simulink model "Adddata_Model"  (R2023a)
settings: Solver=VariableStepAuto  StartTime=0.0  StopTime=10.0  RelTol=1e-3
libraries: NSA_DEVS_SINKS_ATOMIC x6, TimeSharedLib x3, NSA_DEVS_LOGISTICS_ATOMIC x2, NSA_DEVS_SOURCES_ATOMIC x1
settings Model: Creator=david  LastModifiedBy=peter

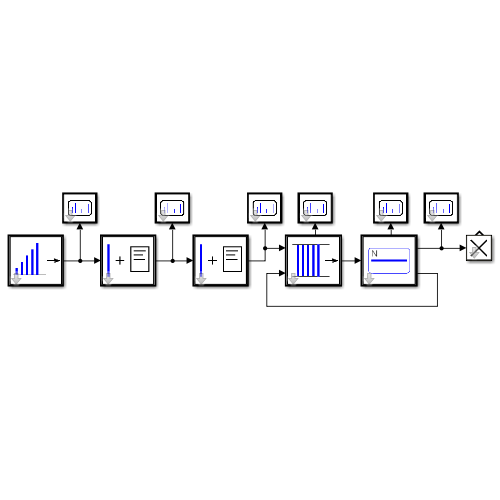
[thumbnail: Simulink's stored preview of the top-level diagram]
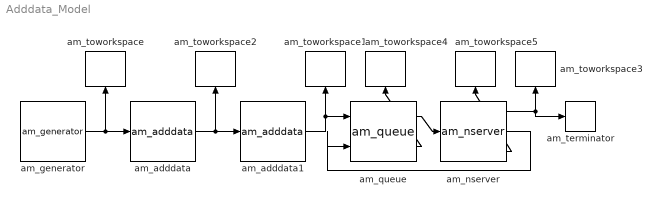
== system Adddata_Model ==
  am_adddata : TimeSharedLib/am_adddata  fields="[\"name\", \"age\"]"  values="[\"Krull\", \"36\"]"  numeric=[false, true]  infield="\"id\""  tau=[0,1]  debug=0
  am_adddata1 : TimeSharedLib/am_adddata  fields="[\"firstname\", \"weight\"]"  values="[\"Felix\", \"73\"]"  numeric=[false, true]  infield="\"id\""  tau=[0,1]  debug=0
  am_generator : NSA_DEVS_SOURCES_ATOMIC/am_generator  tG=1  n0=1  nG=6  tau=[0,1]  debug=0
      settings: SourceProductName=NSA_DEVS
  am_nserver : TimeSharedLib/am_nserver  tS=4.5  N=3  tD=[0,2]  tau=[0,1]  debug=0
  am_queue : NSA_DEVS_LOGISTICS_ATOMIC/am_queue  tD=[0,2]  tau=[0,1]  debug=0
      settings: SourceProductName=NSA_DEVS
  am_terminator : NSA_DEVS_LOGISTICS_ATOMIC/am_terminator  tau=[0,1]  debug=0
      settings: SourceProductName=NSA_DEVS
  am_toworkspace : NSA_DEVS_SINKS_ATOMIC/am_toworkspace  varname="\"genOut\""  t0=0  format="\"vector\""  tau=[0,3]  debug=0
      settings: SourceProductName=NSA_DEVS
  am_toworkspace1 : NSA_DEVS_SINKS_ATOMIC/am_toworkspace  varname="\"data2Out\""  t0=0  format="\"vector\""  tau=[0,3]  debug=0
      settings: SourceProductName=NSA_DEVS
  am_toworkspace2 : NSA_DEVS_SINKS_ATOMIC/am_toworkspace  varname="\"data1Out\""  t0=0  format="\"vector\""  tau=[0,3]  debug=0
      settings: SourceProductName=NSA_DEVS
  am_toworkspace3 : NSA_DEVS_SINKS_ATOMIC/am_toworkspace  varname="\"srv2Out\""  t0=0  format="\"vector\""  tau=[0,3]  debug=0
      settings: SourceProductName=NSA_DEVS
  am_toworkspace4 : NSA_DEVS_SINKS_ATOMIC/am_toworkspace  varname="\"nqOut\""  t0=0  format="\"vector\""  tau=[0,3]  debug=0
      settings: SourceProductName=NSA_DEVS
  am_toworkspace5 : NSA_DEVS_SINKS_ATOMIC/am_toworkspace  varname="\"nsOut\""  t0=0  format="\"vector\""  tau=[0,5]  debug=0
      settings: SourceProductName=NSA_DEVS
  wires:
  am_generator/1 -> am_adddata/1, am_toworkspace/1
  am_adddata1/1 -> am_queue/1, am_toworkspace1/1
  am_adddata/1 -> am_toworkspace2/1, am_adddata1/1
  am_nserver/1 -> am_toworkspace3/1, am_terminator/1
  am_queue/1 -> am_nserver/1
  am_queue/2 -> am_toworkspace4/1
  am_nserver/3 -> am_toworkspace5/1
  am_nserver/2 -> am_queue/2
